simulink model "M04_LQR_SmartThrottle"  (R2025b)
settings: Solver=ode4  StartTime=0.01  StopTime=t_sim_stop  RelTol=1e-3
undefined symbols (not defined in the file): a, b, curvature_array, g, K_array, Kv, L, mass, max_straight_speed, mu, path_waypoints, V_nodes, v_ref_array
libraries: simulink x2, autolibshared x1
settings Model: Creator=Legion  LastModifiedBy=Legion

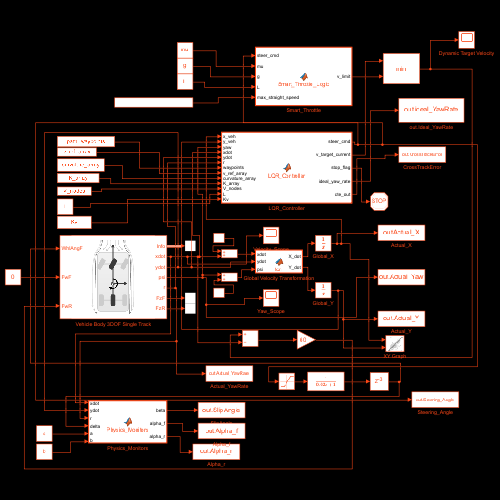
[thumbnail: Simulink's stored preview of the top-level diagram]
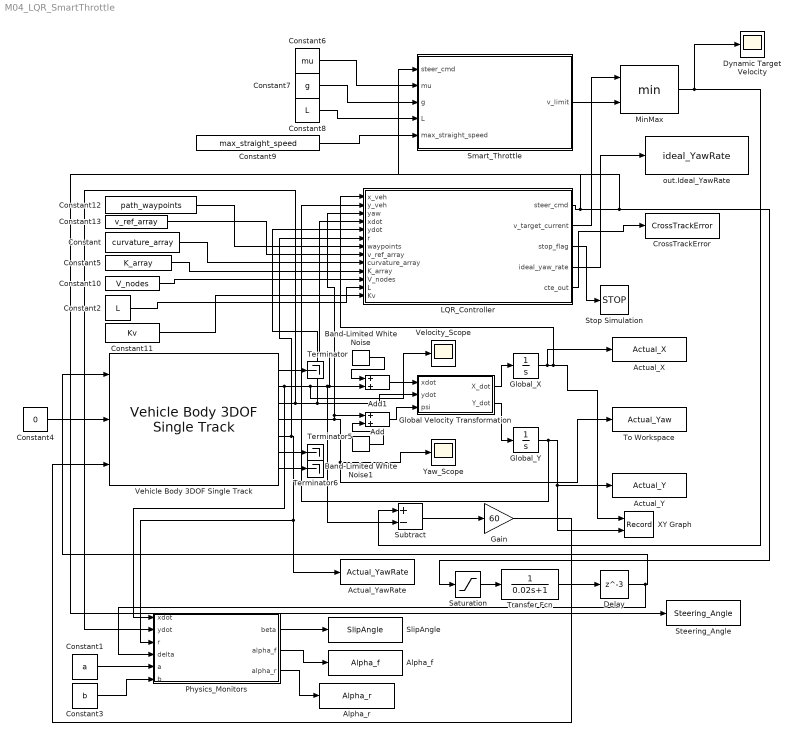
== system M04_LQR_SmartThrottle ==
  Actual_X : ToWorkspace  VariableName=Actual_X  SaveFormat=Timeseries  SampleTime=-1
  Actual_Y : ToWorkspace  VariableName=Actual_Y  SaveFormat=Timeseries  SampleTime=-1
  Actual_YawRate : ToWorkspace  VariableName=Actual_YawRate  SaveFormat=Timeseries  SampleTime=-1
  Add : Sum
  Add1 : Sum
  Alpha_f : ToWorkspace  VariableName=Alpha_f  SaveFormat=Timeseries  SampleTime=-1
  Alpha_r : ToWorkspace  VariableName=Alpha_r  SaveFormat=Timeseries  SampleTime=-1
  Band-Limited White Noise : simulink/Sources/Band-Limited White Noise  Cov=[0.0001]  Ts=0.01  seed=[23341]
  Band-Limited White Noise1 : simulink/Sources/Band-Limited White Noise  Cov=[0.0005]  Ts=0.01  seed=[23341]
  Constant : Constant  Value=curvature_array
  Constant1 : Constant  Value=a
  Constant10 : Constant  Value=V_nodes
  Constant11 : Constant  Value=Kv
  Constant12 : Constant  Value=path_waypoints
  Constant13 : Constant  Value=v_ref_array
  Constant2 : Constant  Value=L
  Constant3 : Constant  Value=b
  Constant4 : Constant  Value=0
  Constant5 : Constant  Value=K_array
  Constant6 : Constant  Value=mu
  Constant7 : Constant  Value=g
  Constant8 : Constant  Value=L
  Constant9 : Constant  Value=max_straight_speed
  CrossTrackError : ToWorkspace  VariableName=CrossTrackError  SaveFormat=Timeseries  SampleTime=-1
  Delay : Delay  DelayLength=3
  Dynamic Target Velocity : Scope
      settings: DataLoggingVariableName=ScopeData2
  Gain : Gain  Gain=60
  Global Velocity Transformation : MATLAB Function  TreatAsAtomicUnit=on
  Global_X : Integrator  InitialCondition=path_waypoints(1,1)
  Global_Y : Integrator  InitialCondition=path_waypoints(1,2)
  LQR_Controller : MATLAB Function  TreatAsAtomicUnit=on
  MinMax : MinMax  Inputs=2
  Physics_Monitors : MATLAB Function  TreatAsAtomicUnit=on
  Saturation : Saturate  UpperLimit=30 * pi/180  LowerLimit=-30 * pi/180
  SlipAngle : ToWorkspace  VariableName=SlipAngle  SaveFormat=Timeseries  SampleTime=-1
  Smart_Throttle : MATLAB Function  TreatAsAtomicUnit=on
  Steering_Angle : ToWorkspace  VariableName=Steering_Angle  SaveFormat=Timeseries  SampleTime=-1
  Stop Simulation : Stop
  Subtract : Sum  Inputs=+-
  Terminator : Terminator
  Terminator5 : Terminator
  Terminator6 : Terminator
  To Workspace : ToWorkspace  VariableName=Actual_Yaw  SaveFormat=Timeseries  SampleTime=-1
  Transfer Fcn : TransferFcn  Denominator=[0.02 1]
  Vehicle Body 3DOF Single Track : autolibshared/Vehicle Body 3DOF Single Track  trackMode=Single (bicycle)  inputMode=External longitudinal forces  frontSteerMode=on  rearSteerMode=off  windMode=off  muMode=off  extFMode=off  extMMode=off  htchFMode=off  htchMMode=off  extXo=off  extpsio=off  extxdoto=off  extro=off  extYo=off  extTamb=off  extydoto=off  aMode=2  NF=2  NR=2  m=mass  a=a  b=b  h=h  dh=1  hh=0.2  X_o=0  xdot_o=0.001  CalphaMode=off  sigmaMode=off  d=0  hl=0  w=[1.4,1.4]  Cy_f=Cy_f  Cy_r=Cy_r  sigma_f=.1  sigma_r=.1  alpha_f_brk=[-0.785, -0.628, -0.471, -0.314, -0.157, 0.000, 0.157, 0.314, 0.471, 0.628, 0.785]  Cy_f_data=[2000, 3000, 4000, 5500, 7000, 9000, 7000, 5500, 4000, 3000, 2000]  alpha_r_brk=[-0.785, -0.628, -0.471, -0.314, -0.157, 0.000, 0.157, 0.314, 0.471, 0.628, 0.785]  Cy_r_data=[2000, 3000, 4000, 5500, 7000, 9000, 7000, 5500, 4000, 3000, 2000]  Y_o=0  ydot_o=0  Izz=Izz  psi_o=atan2(path_waypoints(2,2)-path_waypoints(1,2), path_waypoints(2,1)-path_waypoints(1,1))  r_o=0  Af=Af  Cd=.3  Cl=.1  Cpm=.1  beta_w=[0 0.01:0.01:0.3]  Cs=[0 0.01:0.01:0.3]  Cym=[0 1e-6:0.01:0.3]  Pabs=101325  Tair=273  g=9.81  mu=mu  xdot_tol=.01  Fznom=Fznom  Fxtire_sat=7e4  Fytire_sat=7e4  longOff=0  latOff=0  vertOff=0  wrapAng=off
  Velocity_Scope : Scope
      settings: ActiveDisplayYMinimum=0.7024131164666485  ActiveDisplayYMaximum=1.4316639746586821
  XY Graph : Record  NumPorts=2.0  FileSettingsInternal="{\"entries\":[{\"content\":{\"excelSettings\":{\"content\":{},\"type\":\"Streamout.ExcelSettings\"},\"parquetSettings\":{\"content\":{},\"type\":\"Streamout.ParquetSettings\"}},\"type\":\"Streamout.FileSettingStorage\",\"uuid\":\"\"}],\"packageUris\":[\"http:\\/\\/schema.mathworks.com\\/mf0\\/streamout_blocks\\/R2020a\"],\"version\":\"1.0\"}"  FrameSettings=[0, 0]  Layout=[1 1]  SignalsInternal="{\"entries\":[{\"content\":{\"signals\":[{\"content\":{\"blockPath\":[],\"dimensions\":[1],\"domain\":\"\",\"lineColor\":\"#0072bd\",\"lineWidth\":2,\"port\":1,\"sid\":[\"\"],\"signalID\":1,\"signalName\":\"Global_X\"},\"type\":\"RecordBlkView.Signal\",\"uuid\":\"\"},{\"content\":{\"blockPath\":[],\"dimensions\":[1],\"domain\":\"\",\"lineColor\":\"#d95319\",\"lineWidth\":2,\"port\":2,\"sid\":[\"\"],\"signalID\":2,\"signalName\":\"Global_Y\"},\"type\":\"RecordBlkView.Signal\",\"uuid\":\"\"}]},\"type\":\"RecordBlkView.InputSignals\",\"uuid\":\"\"}],\"packageUris\":[\"http:\\/\\/schema.mathworks.com\\/mf0\\/streamout_blocks\\/R2020a\"],\"version\":\"1.0\"}"  VisualizationBindings="{\"xyplotplugin\":{\"info\":[{\"series\":[],\"subplotID\":1}]}}"  CompatibilityTag=XY
  Yaw_Scope : Scope
      settings: ActiveDisplayYMinimum=-0.24426851447788056  ActiveDisplayYMaximum=1.1237341178679363
  out.Ideal_YawRate : ToWorkspace  VariableName=ideal_YawRate  SaveFormat=Timeseries  SampleTime=-1
  wires:
  Subtract/1 -> Gain/1
  Gain/1 -> Vehicle Body 3DOF Single Track/3
  Vehicle Body 3DOF Single Track/3 -> Global Velocity Transformation/2(ydot), LQR_Controller/5(ydot), Physics_Monitors/2(ydot)
  Vehicle Body 3DOF Single Track/7 -> Terminator6/1
  Saturation/1 -> Transfer Fcn/1
  Vehicle Body 3DOF Single Track/1 -> Terminator/1
  Vehicle Body 3DOF Single Track/4 -> Yaw_Scope/1, To Workspace/1, Add/1, LQR_Controller/3(yaw)
  Global Velocity Transformation/2(Y_dot) -> Global_Y/1
  Transfer Fcn/1 -> Delay/1
  Global_Y/1 -> LQR_Controller/2(y_veh), XY Graph/2, Actual_Y/1
  Global Velocity Transformation/1(X_dot) -> Global_X/1
  Global_X/1 -> Actual_X/1, LQR_Controller/1(x_veh), XY Graph/1
  Constant4/1 -> Vehicle Body 3DOF Single Track/2
  Vehicle Body 3DOF Single Track/6 -> Terminator5/1
  Vehicle Body 3DOF Single Track/5 -> LQR_Controller/6(r), Physics_Monitors/3(r), Actual_YawRate/1
  LQR_Controller/1(steer_cmd) -> Smart_Throttle/1(steer_cmd), Steering_Angle/1, Saturation/1
  Constant2/1 -> LQR_Controller/12(L)
  Constant6/1 -> Smart_Throttle/2(mu)
  Constant7/1 -> Smart_Throttle/3(g)
  Constant8/1 -> Smart_Throttle/4(L)
  Vehicle Body 3DOF Single Track/2 -> Physics_Monitors/1(xdot), Velocity_Scope/1, Add1/2, LQR_Controller/4(xdot), Subtract/2
  MinMax/1 -> Subtract/1, Dynamic Target Velocity/1
  Constant9/1 -> Smart_Throttle/5(max_straight_speed)
  Physics_Monitors/2(alpha_f) -> Alpha_f/1
  Constant1/1 -> Physics_Monitors/5(a)
  Physics_Monitors/1(beta) -> SlipAngle/1
  Physics_Monitors/3(alpha_r) -> Alpha_r/1
  Constant3/1 -> Physics_Monitors/6(b)
  Constant/1 -> LQR_Controller/9(curvature_array)
  Constant5/1 -> LQR_Controller/10(K_array)
  Constant10/1 -> LQR_Controller/11(V_nodes)
  Constant11/1 -> LQR_Controller/13(Kv)
  Constant12/1 -> LQR_Controller/7(waypoints)
  Constant13/1 -> LQR_Controller/8(v_ref_array)
  LQR_Controller/3(stop_flag) -> Stop Simulation/1
  LQR_Controller/2(v_target_current) -> MinMax/1
  Smart_Throttle/1(v_limit) -> MinMax/2
  LQR_Controller/4(ideal_yaw_rate) -> out.Ideal_YawRate/1
  Add/1 -> Global Velocity Transformation/3(psi)
  Add1/1 -> Global Velocity Transformation/1(xdot)
  Band-Limited White Noise/1 -> Add1/1
  Band-Limited White Noise1/1 -> Add/2
  Delay/1 -> Physics_Monitors/4(delta), Vehicle Body 3DOF Single Track/1
  LQR_Controller/5(cte_out) -> CrossTrackError/1

== matlab function M04_LQR_SmartThrottle/Physics_Monitors ==
  data: xdot input; beta output; ydot input; r input; delta input; a input; b input; alpha_f output; alpha_r output
function [beta, alpha_f, alpha_r] = Physics_Monitors(xdot, ydot, r, delta, a, b)
    % This block mathematically derives the slip angles to prove tire saturation.
    % xdot: Longitudinal velocity (m/s)
    % ydot: Lateral velocity (m/s)
    % r: Yaw rate (rad/s)
    % delta: Actual front wheel steering angle (rad)
    % a, b: Distances from CG to front/rear axles (m)

    % 1. Safety limit to prevent division by zero when starting from a standstill
    v_x_safe = max(xdot, 0.1); 

    % 2. Vehicle Slip Angle (\beta)
    % Angle between the vehicle's longitudinal axis and its actual direction of travel
    beta = atan(ydot / v_x_safe);

    % 3. Front Tire Slip Angle (\alpha_f)
    % Combines lateral velocity, yaw rotation effect (a*r), and subtracts steering angle
    alpha_f = atan((ydot + a * r) / v_x_safe) - delta;

    % 4. Rear Tire Slip Angle (\alpha_r)
    % Combines lateral velocity and yaw rotation effect (rear axle moves opposite to front during yaw)
    alpha_r = atan((ydot - b * r) / v_x_safe);
end

== matlab function M04_LQR_SmartThrottle/Global Velocity Transformation ==
  data: xdot input; X_dot output; ydot input; psi input; Y_dot output
function [X_dot, Y_dot] = fcn(xdot, ydot, psi)
    % Rotate Body Velocities into Global Map Velocities
    X_dot = xdot * cos(psi) - ydot * sin(psi);
    Y_dot = xdot * sin(psi) + ydot * cos(psi);
end

== matlab function M04_LQR_SmartThrottle/LQR_Controller ==
  settings: updateMethod=DISCRETE  sampleTime=0.01
  data: x_veh input; steer_cmd output; y_veh input; yaw input; xdot input; ydot input; r input; waypoints input; v_ref_array input; curvature_array input; K_array input; V_nodes input; L input; Kv input; v_target_current output; stop_flag output; ideal_yaw_rate output; cte_out output
function [steer_cmd, v_target_current, stop_flag, ideal_yaw_rate, cte_out] = LQR_Controller(x_veh, y_veh, yaw, xdot, ydot, r, waypoints, v_ref_array, curvature_array, K_array, V_nodes, L, Kv)
    persistent has_finished last_closest_idx;
    if isempty(has_finished), has_finished = false; end
    if isempty(last_closest_idx), last_closest_idx = 1; end
    stop_flag = 0;
    
    % 1. Finish Line Logic
    if last_closest_idx > (length(waypoints) * 0.95)
        dx_track = waypoints(end, 1) - waypoints(end-1, 1);
        dy_track = waypoints(end, 2) - waypoints(end-1, 2);
        dx_car = x_veh - waypoints(end, 1);
        dy_car = y_veh - waypoints(end, 2);
        if (dx_track * dx_car + dy_track * dy_car) > 0, has_finished = true; end
    end
    if has_finished
        steer_cmd = 0; v_target_current = 0; stop_flag = 1; ideal_yaw_rate = 0; cte_out = 0; return;
    end
    
    % 2. Find Closest Waypoint & VELOCITY LOOKAHEAD (0.6s)
    min_dist = inf; closest_idx = last_closest_idx;
    for i = last_closest_idx:(size(waypoints, 1) - 1)
        d = sqrt((waypoints(i,1) - x_veh)^2 + (waypoints(i,2) - y_veh)^2);
        if d < min_dist
            min_dist = d; closest_idx = i;
        end
    end
    last_closest_idx = closest_idx; 
    
    lookahead_time = 0.6; 
    lookahead_dist = max(xdot, 1.0) * lookahead_time;
    idx_offset = round(lookahead_dist / 0.05); 
    target_idx = min(size(waypoints, 1), closest_idx + idx_offset);
    
    v_target_current = v_ref_array(target_idx);
    
    % 3. Calculate Path Kinematics
    dx = waypoints(closest_idx+1, 1) - waypoints(closest_idx, 1);
    dy = waypoints(closest_idx+1, 2) - waypoints(closest_idx, 2);
    yaw_path = atan2(dy, dx);
    kappa = curvature_array(closest_idx); 
    
    % 4. State Vector Formulation [e, e_dot, theta_e, theta_e_dot]
    l2 = dx^2 + dy^2;
    if l2 > 0
        t = ((x_veh - waypoints(closest_idx, 1)) * dx + (y_veh - waypoints(closest_idx, 2)) * dy) / l2;
        proj_x = waypoints(closest_idx, 1) + t * dx;
        proj_y = waypoints(closest_idx, 2) + t * dy;
    else
        proj_x = waypoints(closest_idx, 1); proj_y = waypoints(closest_idx, 2);
    end
    e_mag = sqrt((x_veh - proj_x)^2 + (y_veh - proj_y)^2);
    cross_prod = dx * (y_veh - waypoints(closest_idx, 2)) - dy * (x_veh - waypoints(closest_idx, 1));
    
    e = sign(cross_prod) * e_mag;
    
    theta_e = yaw - yaw_path;
    theta_e = atan2(sin(theta_e), cos(theta_e)); 
    
    e_dot = ydot + xdot * sin(theta_e);
    
    yaw_rate_path = kappa * xdot;
    ideal_yaw_rate = yaw_rate_path; 
    theta_e_dot = r - yaw_rate_path;
    
    % 5. Linear Quadratic Regulator (LQR) Feedback
    v_safe = max(xdot, 1.0); 
    K = [interp1(V_nodes, K_array(:,1), v_safe, 'linear', 'extrap'), ...
         interp1(V_nodes, K_array(:,2), v_safe, 'linear', 'extrap'), ...
         interp1(V_nodes, K_array(:,3), v_safe, 'linear', 'extrap'), ...
         interp1(V_nodes, K_array(:,4), v_safe, 'linear', 'extrap')];
         
    steer_feedback = - (K(1)*e + K(2)*e_dot + K(3)*theta_e + K(4)*theta_e_dot);
    
    % 6. Feedforward Control 
    steer_feedforward = (kappa * L) + (kappa * Kv * v_safe^2);
    
    % 7. Final Command & Saturation
    steer_cmd = steer_feedback + steer_feedforward;
    steer_max = 30 * (pi/180);
    cte_out = e;
    if steer_cmd > steer_max, steer_cmd = steer_max;
    elseif steer_cmd < -steer_max, steer_cmd = -steer_max; end
end

== matlab function M04_LQR_SmartThrottle/Smart_Throttle ==
  settings: updateMethod=DISCRETE  sampleTime=0.01
  data: steer_cmd input; v_limit output; mu input; g input; L input; max_straight_speed input
function v_limit = Smart_Throttle_Logic(steer_cmd, mu, g, L, max_straight_speed)
    persistent v_prev;
    if isempty(v_prev)
        v_prev = max_straight_speed; 
    end
    
    margin = 0.85; 
    abs_steer = abs(steer_cmd); 
    
    % 5-Degree Deadband (0.087 radians)
    if abs_steer < 0.087 
        v_raw = max_straight_speed;
    else
        R_curve = L / tan(abs_steer);
        v_raw = sqrt(mu * g * abs(R_curve)) * margin;
    end
    
    % Asymmetric Smoothing
    if v_raw < v_prev
        % Braking: Smooth and gradual to keep weight transfer stable
        alpha = 0.15; 
    else
        % Accelerating: Snap the throttle open immediately!
        alpha = 0.80; 
    end
    
    v_filtered = (alpha * v_raw) + (1 - alpha) * v_prev;
    v_prev = v_filtered;
    
    v_limit = min(v_filtered, max_straight_speed); 
end
